simulink model "frekvens"  (R2017b)
settings: Solver=VariableStepAuto  StartTime=-5  StopTime=120  RelTol=1e-3
values from neighbouring files (symbols this model uses):
  J = Ponline*H/(wnom^2/2)    [initfrek.m]
  Pref = Pe-PDCfref=f    [initfrek.m]
  Pt = Pe-PDCPonline=1.2*PtH=3.6    [initfrek.m]
  R = 20e9    (= 20000000000)    [initfrek.m]
undefined symbols (not defined in the file or in its folder): D, fref, K, PDC, wnom
settings Model: Creator=ielolof  LastModifiedBy=ielolof

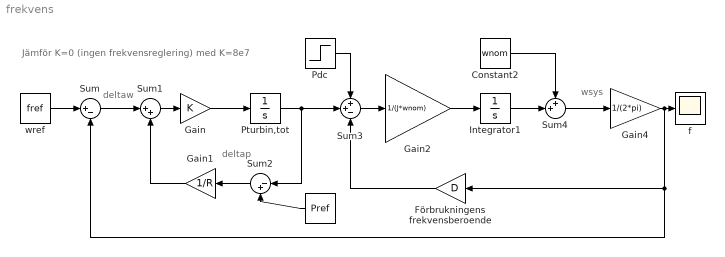
== system frekvens ==
  note: Jämför K=0 (ingen frekvensreglering) med K=8e7
  note: wsys
  note: deltap
  note: deltaw
  " " : Constant  Value=Pref
  Constant2 : Constant  Value=wnom
  Förbrukningens frekvensberoende : Gain  Gain=D
  Gain : Gain  Gain=K
  Gain1 : Gain  Gain=1/R
  Gain2 : Gain  Gain=1/(J*wnom)
  Gain4 : Gain  Gain=1/(2*pi)
  Integrator1 : Integrator
  Pdc : Step  Time=0  Before=PDC  After=0  SampleTime=0
  Pturbin,tot : Integrator  InitialCondition=Pt
  Sum : Sum  Inputs=|+-
  Sum1 : Sum  Inputs=|++
  Sum2 : Sum  Inputs=|-+
  Sum3 : Sum  Inputs=++-
  Sum4 : Sum  Inputs=++|
  f : Scope
  wref : Constant  Value=fref
  wires:
  wref/1 -> Sum/1
  Sum/1 -> Sum1/1
  Sum1/1 -> Gain/1
  Gain/1 -> Pturbin,tot/1
  Pturbin,tot/1 -> Sum2/1, Sum3/2
  Sum3/1 -> Gain2/1
  Gain2/1 -> Integrator1/1
  Integrator1/1 -> Sum4/2
  Pdc/1 -> Sum3/1
  Förbrukningens frekvensberoende/1 -> Sum3/3
  Sum4/1 -> Gain4/1
  Constant2/1 -> Sum4/1
  " "/1 -> Sum2/2
  Sum2/1 -> Gain1/1
  Gain1/1 -> Sum1/2
  Gain4/1 -> Förbrukningens frekvensberoende/1, Sum/2, f/1
